simulink model "motorcontrol_codegen_19a"  (R2019a)
settings: Solver=FixedStepDiscrete  StartTime=0.0  StopTime=Inf  MaxStep=5e-5  RelTol=1e-3  EnableMultiTasking=on
values from neighbouring files (symbols this model uses):
  dataType = 'single'    [motorcontrol_codegen_params.m]
undefined symbols (not defined in the file or in its folder): ControlMode, ctrlParams, DiscIntNeverNeededParam, Down, GPTRIP1SEL, GPTRIP2SEL, inverter, mcb_isSimVar, NumBits1, NumBits2, PI_params, pmsm, Slope1, Slope2, Target, Ts, TZ1, TZ2, Up
libraries: simulink x14, c2802xlib x5, c2837xDlib x4, c280xlib x1, c2000lib x1
(part 1 of 3)
settings Model: SimulationMode=external  ExtModeTrigDuration=8  Creator=26046633  LastModifiedBy=26046633
settings SolverCC: ZeroCrossAlgorithm=Adaptive
settings OptimizationCC: DefaultUnderspecifiedDataType=single  StateBitsets=on  DataBitsets=on  NoFixptDivByZeroProtection=on  EfficientFloat2IntCast=on  LifeSpan=inf  MaxStackSize=1024  DifferentSizesBufferReuse=on  OptimizationPriority=RAM  DenormalBehavior=FlushToZero
settings DebuggingCC: IgnoredZcDiagnostic=none  MultiTaskDSMMsg=none  IntegerOverflowMsg=none  ParameterOverflowMsg=none  ParameterPrecisionLossMsg=none  ParameterTunabilityLossMsg=error
settings HardwareCC: ProdBitPerChar=16  ProdBitPerInt=16  ProdBitPerPointer=32  ProdBitPerSizeT=32  ProdBitPerPtrDiffT=32  ProdLargestAtomicInteger=Integer  ProdLargestAtomicFloat=None  ProdWordSize=16  ProdLongLongMode=on  ProdHWDeviceType=Texas Instruments->C2000
settings ModelReferenceCC: PropagateSignalLabelsOutOfModel=off
settings SFSimCC: MATLABDynamicMemAlloc=off
settings RTWCC: SystemTargetFile=ert.tlc  HardwareBoard=TI Delfino F2837xD  TLCOptions=-aInlineSetEventsForThisBaseRateFcn=TLC_FALSE -aSuppressMultiTaskScheduler=TLC_FALSE -aRateBasedStepFcn=1  GenCodeOnly=on  TemplateMakefile=ert_default_tmf  Toolchain=Texas Instruments Code Composer Studio (C2000)  PortableWordSizes=on  CreateSILPILBlock=SIL
settings CodeAppCC: ForceParamTrailComments=on  IgnoreCustomStorageClasses=off  OperatorAnnotations=on  SimulinkDataObjDesc=on  SFDataObjDesc=on  CustomSymbolStrGlobalVar=rt$N$M  CustomSymbolStrType=$N$M  CustomSymbolStrFcn=$N$M$F  CustomSymbolStrMacro=$N$M  InsertBlockDesc=on
settings ERTTargetCC: CodeReplacementLibrary=TI C28x  IncludeMdlTerminateFcn=off  CombineSignalStateStructs=on  SupportNonInlinedSFcns=on  ExtModeTransport=3  ExtModeStaticAllocSize=10000  ERTFilePackagingFormat=CompactWithDataFile

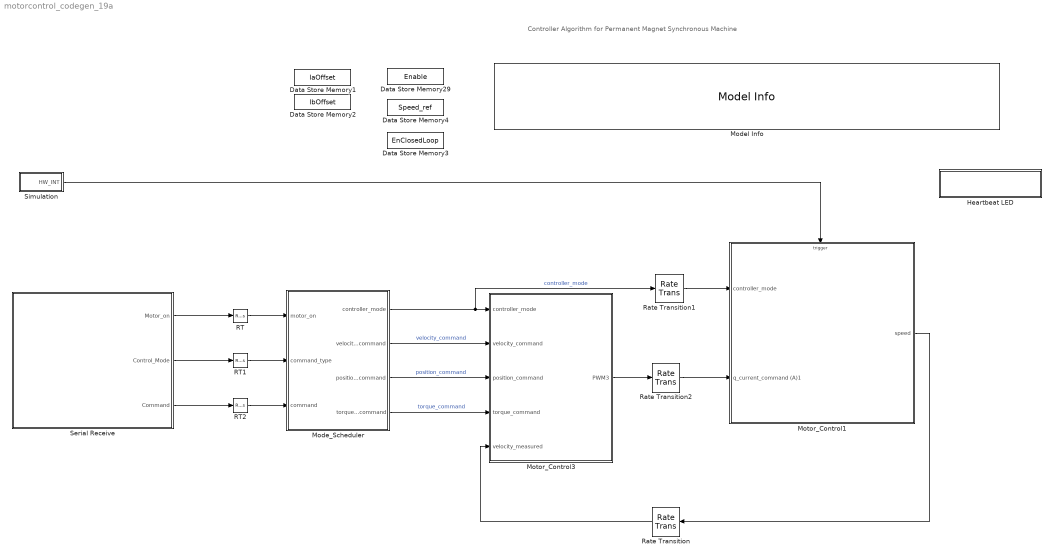
== system motorcontrol_codegen_19a ==
  note: Controller Algorithm for Permanent Magnet Synchronous Machine
  Data Store Memory1 : DataStoreMemory  DataStoreName=IaOffset  InitialValue=inverter.CtSensAOffset  ShowAdditionalParam=off
  Data Store Memory2 : DataStoreMemory  DataStoreName=IbOffset  InitialValue=inverter.CtSensBOffset  ShowAdditionalParam=off
  Data Store Memory29 : DataStoreMemory  DataStoreName=Enable  ShowAdditionalParam=off  OutDataTypeStr=boolean
  Data Store Memory3 : DataStoreMemory  DataStoreName=EnClosedLoop  ShowAdditionalParam=off  OutDataTypeStr=boolean
  Data Store Memory4 : DataStoreMemory  DataStoreName=Speed_ref  ShowAdditionalParam=off  OutDataTypeStr=dataType
  Heartbeat LED : Subsystem  TreatAsAtomicUnit=on
  Mode_Scheduler : Subsystem  TreatAsAtomicUnit=on  SystemSampleTime=Ts.speed
      mask Display: fprintf('Mode\nScheduler')
  Model Info : simulink/Model-Wide Utilities/Model Info  Frame=on  DisplayStringWithTags=|  HorizontalTextAlignment=Left  LeftAlignmentValue=0.02
      | %<Description>  Model Description: Controller Algorithm for Permanent Magnet Synchronous Motor
      | 
      | %<ModifiedComment> Specifies controller software for Permanent Magnet Synchronous Machine (PMSM) using Field-Oriented Control.
      | 
      | Created By: %<Created>  | Alper Senem [26046633]
      | Last Modification: %<LastModificationDate> | %<LastModifiedBy>
      | Version: %<ModelVersion>
  Motor_Control1 : Subsystem
      settings: RTWSystemCode=Nonreusable function
      mask Display: fprintf('Field Oriented\nControl')
  Motor_Control3 : Subsystem  TreatAsAtomicUnit=on  SystemSampleTime=Ts.speed
      settings: RTWSystemCode=Nonreusable function  RTWFcnNameOpts=Use subsystem name
      mask Display: fprintf('Motor\nControl')
  RT : RateTransition  Deterministic=off  OutPortSampleTime=Ts.speed
  RT1 : RateTransition  Integrity=off  Deterministic=off  OutPortSampleTime=Ts.speed
  RT2 : RateTransition  Deterministic=off  OutPortSampleTime=Ts.speed
  Rate Transition : RateTransition  Deterministic=off  OutPortSampleTime=Ts.speed
  Rate Transition1 : RateTransition  Integrity=off  Deterministic=off
  Rate Transition2 : RateTransition  Deterministic=off
  Serial Receive : Subsystem
  Simulation : Subsystem
  wires:
  RT1/1 -> Mode_Scheduler/2(command_type)
  RT2/1 -> Mode_Scheduler/3(command)
  Serial Receive/2(Control_Mode) -> RT1/1
  Rate Transition1/1 -> Motor_Control1/1(controller_mode)
  Motor_Control1/1(speed) -> Rate Transition/1
  Mode_Scheduler/2(velocity_command) -> Motor_Control3/2(velocity_command)  "velocity_command"
  Rate Transition2/1 -> Motor_Control1/2(q_current_command (A)1)
  Mode_Scheduler/3(position_command) -> Motor_Control3/3(position_command)  "position_command"
  Mode_Scheduler/4(torque_command) -> Motor_Control3/4(torque_command)  "torque_command"
  Mode_Scheduler/1(controller_mode) -> Motor_Control3/1(controller_mode), Rate Transition1/1  "controller_mode"
  Serial Receive/1(Motor_on) -> RT/1
  Simulation/1(HW_INT) -> Motor_Control1/Trigger
  Rate Transition/1 -> Motor_Control3/5(velocity_measured)
  RT/1 -> Mode_Scheduler/1(motor_on)
  Serial Receive/3(Command) -> RT2/1
  Motor_Control3/1(PWM3) -> Rate Transition2/1

== system motorcontrol_codegen_19a/Heartbeat LED ==
  note: Heartbeat LED 1HZ
  RED_LED : Constant  OutDataTypeStr=uint16  SampleTime=0.1
  Subsystem : Subsystem
  wires:
  RED_LED/1 -> Subsystem/1(In1)

== system motorcontrol_codegen_19a/Mode_Scheduler ==
  note: Mode Scheduler
  note: Configures controller mode and controller inputs based on user commands.
  motor_on : Inport
  command_type : Inport  Port=2
  command : Inport  Port=3
  Controller_Mode_Scheduler : Stateflow chart  SystemSampleTime=Ts
  Signal Conversion : SignalConversion  OverrideOpt=on
  Signal Conversion1 : SignalConversion  OverrideOpt=on
  Signal Conversion2 : SignalConversion  OverrideOpt=on
  controller_mode : Outport
  velocity_command : Outport  Port=2
  position_command : Outport  Port=3
  torque_command : Outport  Port=4
  wires:
  Signal Conversion2/1 -> Controller_Mode_Scheduler/3(command)
  Signal Conversion1/1 -> Controller_Mode_Scheduler/2(command_type)
  Signal Conversion/1 -> Controller_Mode_Scheduler/1(motor_on)
  command/1 -> Signal Conversion2/1
  Controller_Mode_Scheduler/4(torque_command) -> torque_command/1
  command_type/1 -> Signal Conversion1/1
  Controller_Mode_Scheduler/3(position_command) -> position_command/1
  motor_on/1 -> Signal Conversion/1
  Controller_Mode_Scheduler/2(velocity_command) -> velocity_command/1
  Controller_Mode_Scheduler/1(controller_mode) -> controller_mode/1

== system motorcontrol_codegen_19a/Motor_Control1 ==
  note: Field Oriented Controller
  note: This layer executes the control law, and calculates compare values used by the PWM driver.
      | The controller outputs compare values used by the Pulse Width Modulators (PWMs) to generate the phase voltages.
  controller_mode : Inport
  q_current_command (A)1 : Inport  Port=2
  Trigger : TriggerPort  TriggerType=function-call  VariantControl=Variant  SampleTime=-1  PortDimensions=1
  ControlSystem : Subsystem
  Demux1 : Demux
  Input Scaling : Subsystem
  "Inverter " : Subsystem
  Mux : Mux  Inputs=2
  Output Scaling : Subsystem
  Sensor Driver Blocks : Subsystem  VariantControl=mcb_isSimVar()
  speed : Outport
  wires:
  ControlSystem/1(Vabc) -> Output Scaling/1(Vabc_ref)
  Demux1/4 -> Input Scaling/4(QEP_Index_Latch)
  Output Scaling/2(PWM_Enable) -> Mux/2
  Input Scaling/3(EnClosedLoop) -> ControlSystem/5(EnClosedLoop)
  q_current_command (A)1/1 -> ControlSystem/2(q_current_command (A)1)
  Sensor Driver Blocks/1(Out) -> Demux1/1
  Input Scaling/2(Iab_meas) -> ControlSystem/4(Iab_fb)  "Iab_fb"
  Demux1/1 -> Input Scaling/1(Ia_ADC)
  Input Scaling/1(Pos) -> ControlSystem/3(Pos)  "Position"
  Input Scaling/4(speed) -> ControlSystem/6(speed), speed/1  "Speed"
  controller_mode/1 -> ControlSystem/1(controller_mode)
  Demux1/2 -> Input Scaling/2(Ib_ADC)
  Demux1/3 -> Input Scaling/3(QEP_Position_Count)
  Output Scaling/1(PWM_Duty_Cycles) -> Mux/1
  Mux/1 -> "Inverter "/1(Inverter Signals)

== system motorcontrol_codegen_19a/Motor_Control3 ==
  note: This layer executes the control law, and calculates compare values used by the PWM driver.
      | The controller outputs compare values used by the Pulse Width Modulators (PWMs) to generate the phase voltages.
  note: Motor Control
  controller_mode : Inport
  velocity_command : Inport  Port=2
  position_command : Inport  Port=3
  torque_command : Inport  Port=4
  velocity_measured : Inport  Port=5
  Control Modes : Subsystem
  Ground : Ground
  Rate Transition : RateTransition  Deterministic=off  OutPortSampleTime=Ts.speed
  Subsystem1 : Subsystem  mask{FilterConstant=0.01*(Ts.speed/Ts.pwm)}
      mask prompts: FilterConstant "Filter coefficient"
      mask help:
      | Implement an IIR Filter on target hardware by implementing the formula:
      |
      |  y_k = a.x_k + (1-a).y_(k-1)
      |
      | Where, a is the filter coefficient.
      | Lower filter coefficient gives better filtering, but increases the delay in response time.
      mask TypeOptions FilterConstant: Filter_Constant/Value
      mask DialogControl DescGroupVar Prompt: IIR Filter
      mask DialogControl DescTextVar Prompt: Implement an IIR Filter on target hardware by implementing the formula:   y_k = a.x_k + (1-a).y_(k-1)  Where, a is the filter coefficient. Lower filter coefficient gives better filtering, but increases the delay in response time.
      mask Display: fprintf('IIR\n Filter')
  Subsystem2 : Subsystem
  PWM3 : Outport
  wires:
  controller_mode/1 -> Control Modes/1(controller_mode)
  Control Modes/1(PWM3) -> PWM3/1
  Rate Transition/1 -> Control Modes/6(position_measured)
  position_command/1 -> Control Modes/5(position_command)
  torque_command/1 -> Control Modes/4(torque_command)
  Subsystem1/1(y) -> Control Modes/2(velocity_command)  "Speed_ref"
  velocity_command/1 -> Subsystem2/1(Speed_Ref_In)
  Subsystem2/1(Speed_Ref_PU) -> Subsystem1/1(x)  "Speed_Ref"
  velocity_measured/1 -> Subsystem2/2(Speed_Ref_Open), Control Modes/3(velocity_measured)  "Speed_fb"
  Ground/1 -> Rate Transition/1

== system motorcontrol_codegen_19a/Serial Receive ==
  Command_Type : simulink/Sources/Enumerated Constant  OutDataTypeStr=Enum: ControlMode  Value=ControlMode.Speed  SampleTime=-1
  Data Store Write : DataStoreWrite  DataStoreName=Enable
  Data Store Write1 : DataStoreWrite  DataStoreName=Speed_ref
  Data_Type_Float : Subsystem  VariantControl=isequal(dataType, 'single')
  Simulation : Subsystem
  unParse : Subsystem
  Motor_on : Outport
  Control_Mode : Outport  Port=2
  Command : Outport  Port=3
  wires:
  Data_Type_Float/1(Desired Speed) -> Data Store Write1/1, Command/1  "Command"
  Command_Type/1 -> Control_Mode/1  "Control_Mode"
  unParse/1(Enable_PWM) -> Motor_on/1, Data Store Write/1
  Data_Type_Float/2(Out2) -> unParse/1(Data)
  Simulation/1(Data) -> Data_Type_Float/1(Data)

== system motorcontrol_codegen_19a/Simulation ==
  C28x Hardware Interrupt : c2000lib/Scheduling/C28x Hardware Interrupt  irqnumbers=1  pienumbers=2  irqpriorities=30  irqpreempts=1  showinput=off  dspchiptype=C280X
      settings: SourceProductName=Embedded Coder Support Package for Texas Instruments C2000 Processors
  HW_INT : Outport
  wires:
  C28x Hardware Interrupt/1 -> HW_INT/1

== system motorcontrol_codegen_19a/Heartbeat LED/Subsystem ==
  In1 : Inport
  Digital Output : c2837xDlib/Digital Output  GPIO_Number=GPIO32~GPIO39  GPIO_Bit0=off  GPIO_BIT0_Toggle=on  GPIO_Bit1=off  GPIO_BIT1_Toggle=off  GPIO_Bit2=on  GPIO_BIT2_Toggle=on  GPIO_Bit3=off  GPIO_BIT3_Toggle=off  GPIO_Bit4=off  GPIO_BIT4_Toggle=off  GPIO_Bit5=off  GPIO_BIT5_Toggle=off  GPIO_Bit6=off  GPIO_BIT6_Toggle=off  GPIO_Bit7=off  GPIO_BIT7_Toggle=off
      settings: SourceProductName=Embedded Coder Support Package for Texas Instruments C2000 Processors
  wires:
  In1/1 -> Digital Output/1

== system motorcontrol_codegen_19a/Motor_Control1/ControlSystem ==
  controller_mode : Inport
  q_current_command (A)1 : Inport  Port=2
  Pos : Inport  Port=3
  Iab_fb : Inport  Port=4
  EnClosedLoop : Inport  Port=5
  speed : Inport  Port=6
  Closed_Loop : Subsystem
  NOT : Logic  Operator=NOT  IconShape=distinctive  AllPortsSameDT=off  OutDataTypeStr=boolean
  Open Loop Start-Up : Subsystem
  Switch4 : Switch  Threshold=0.5  OutDataTypeStr=Inherit: Inherit via back propagation  RndMeth=Simplest
  Vabc : Outport
  wires:
  Open Loop Start-Up/1(Vabc) -> Switch4/3
  EnClosedLoop/1 -> Closed_Loop/Enable, Switch4/2, NOT/1
  controller_mode/1 -> Closed_Loop/1(controller_mode)
  q_current_command (A)1/1 -> Closed_Loop/2(q_current_command (A)1)
  Closed_Loop/1(Vabc) -> Switch4/1
  NOT/1 -> Open Loop Start-Up/Enable
  Switch4/1 -> Vabc/1
  Pos/1 -> Closed_Loop/3(Feedback)
  Iab_fb/1 -> Closed_Loop/4(Iab_fb)
  speed/1 -> Closed_Loop/5(Speed)

== system motorcontrol_codegen_19a/Motor_Control1/Input Scaling ==
  note: QEP
  note: Position & Speed Measurements
  note: Current Measurements
  Ia_ADC : Inport
  Ib_ADC : Inport  Port=2
  QEP_Position_Count : Inport  Port=3
  QEP_Index_Latch : Inport  Port=4
  " Calculate Position and Speed" : Subsystem
  Calculate Phase Currents : Subsystem
  IndexOffset : Constant  Value=pmsm.PositionOffset * 2 * pi  OutDataTypeStr=dataType  SampleTime=-1
  Pos : Outport
  Iab_meas : Outport  Port=2
  EnClosedLoop : Outport  Port=3
  speed : Outport  Port=4
  wires:
  " Calculate Position and Speed"/3(IndexFound) -> EnClosedLoop/1
  IndexOffset/1 -> " Calculate Position and Speed"/3(Offset)
  QEP_Index_Latch/1 -> " Calculate Position and Speed"/2(QEP_Index_Latch)
  Ib_ADC/1 -> Calculate Phase Currents/2(Ib_ADC)
  Ia_ADC/1 -> Calculate Phase Currents/1(Ia_ADC)
  " Calculate Position and Speed"/1(Theta_e) -> Pos/1
  QEP_Position_Count/1 -> " Calculate Position and Speed"/1(QEP_Position_Count)
  Calculate Phase Currents/1(Iab_meas) -> Iab_meas/1  "Iab_fb"
  " Calculate Position and Speed"/2(speed) -> speed/1

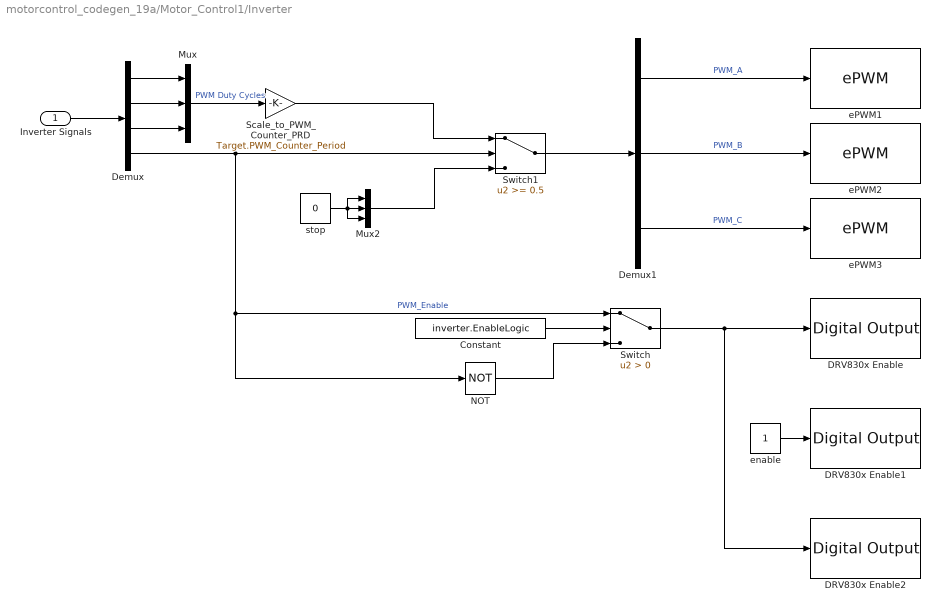
== system motorcontrol_codegen_19a/Motor_Control1/Inverter  ==
  Inverter Signals : Inport
  Constant : Constant  Value=inverter.EnableLogic  SampleTime=-1
  DRV830x Enable : c2837xDlib/Digital Output  GPIO_Number=GPIO40~GPIO47  GPIO_Bit0=on  GPIO_BIT0_Toggle=off  GPIO_Bit1=off  GPIO_BIT1_Toggle=off  GPIO_Bit2=off  GPIO_BIT2_Toggle=off  GPIO_Bit3=off  GPIO_BIT3_Toggle=off  GPIO_Bit4=off  GPIO_BIT4_Toggle=off  GPIO_Bit5=off  GPIO_BIT5_Toggle=off  GPIO_Bit6=off  GPIO_BIT6_Toggle=off  GPIO_Bit7=off  GPIO_BIT7_Toggle=off
      settings: SourceProductName=Embedded Coder Support Package for Texas Instruments C2000 Processors
  DRV830x Enable1 : c2837xDlib/Digital Output  GPIO_Number=GPIO40~GPIO47  GPIO_Bit0=off  GPIO_BIT0_Toggle=off  GPIO_Bit1=on  GPIO_BIT1_Toggle=off  GPIO_Bit2=off  GPIO_BIT2_Toggle=off  GPIO_Bit3=off  GPIO_BIT3_Toggle=off  GPIO_Bit4=off  GPIO_BIT4_Toggle=off  GPIO_Bit5=off  GPIO_BIT5_Toggle=off  GPIO_Bit6=off  GPIO_BIT6_Toggle=off  GPIO_Bit7=off  GPIO_BIT7_Toggle=off
      settings: SourceProductName=Embedded Coder Support Package for Texas Instruments C2000 Processors
  DRV830x Enable2 : c2837xDlib/Digital Output  GPIO_Number=GPIO56~GPIO63  GPIO_Bit0=off  GPIO_BIT0_Toggle=off  GPIO_Bit1=off  GPIO_BIT1_Toggle=off  GPIO_Bit2=on  GPIO_BIT2_Toggle=off  GPIO_Bit3=off  GPIO_BIT3_Toggle=off  GPIO_Bit4=off  GPIO_BIT4_Toggle=off  GPIO_Bit5=off  GPIO_BIT5_Toggle=off  GPIO_Bit6=off  GPIO_BIT6_Toggle=off  GPIO_Bit7=off  GPIO_BIT7_Toggle=off
      settings: SourceProductName=Embedded Coder Support Package for Texas Instruments C2000 Processors
  Demux : Demux
  Demux1 : Demux  Outputs=3
  Mux : Mux  Inputs=3
  Mux2 : Mux  Inputs=3
  NOT : Logic  Operator=NOT  IconShape=distinctive  AllPortsSameDT=off  OutDataTypeStr=boolean
  Scale_to_PWM_Counter_PRD : Gain  Gain=Target.PWM_Counter_Period  OutDataTypeStr=uint16  RndMeth=Simplest
  Switch : Switch  Criteria=u2 > Threshold  OutDataTypeStr=uint16
  Switch1 : Switch  Threshold=0.5
  ePWM1 : c2802xlib/ePWM  PwmType=C2000_Type4  useModule=ePWM1  ePWMxLINKTBPRD=Not Linked  periodUnits=Clock cycles  timerSource=Specify via dialog  timerPeriod_clk=Target.PWM_Counter_Period+1  timerPeriod_sec=0.0001  tbshadow=Immediate without using shadow  countingMode=Up-Down  phaseActiveEnable=Disable  phaseDirection=Count down after sync  phaseActive=0  synchronizationEnable=off  dcaevt1Sync=off  dcbevt1Sync=off  synchronizationOption=Counter equals to zero (CTR=Zero)  perSynchronizationOption=Counter equals to period (CTR=PRD)  clockPrescale=1  HSclockPrescale=1  enswap=off  ePWMxAStatus=on  ePWMxAactionLogic1=Do nothing  ePWMxAactionLogic2=Do nothing  ePWMxAactionLogic3=Clear  ePWMxAactionLogic4=Set  ePWMxAactionLogic5=Do nothing  ePWMxAactionLogic6=Do nothing  ePWMxACSFenable=off  ePWMxACSFvalue=Forcing disable  ePWMxASFreload=Zero  ePWMxBStatus=off  ePWMxBactionLogic1=Do nothing  ePWMxBactionLogic2=Do nothing  ePWMxBactionLogic3=Clear  ePWMxBactionLogic4=Set  ePWMxBactionLogic5=Do nothing  ePWMxBactionLogic6=Do nothing  ePWMxBCSFenable=off  ePWMxBCSFvalue=Forcing disable  ePWMxBSFreload=Zero  ePWNxBOutWay=off  ePWMxLINKCMPA=Not Linked  CMPAUnits=Clock cycles  CMPASource=Input port  CMPAValue_per=50  CMPAValue_clk=floor(Target.PWM_Counter_Period/2+1)  enCMPAshadow=Counter equals to zero (CTR=Zero)  ePWMxLINKCMPB=Not Linked  CMPBUnits=Clock cycles  CMPBSource=Specify via dialog  CMPBValue_per=50  CMPBValue_clk=floor(Target.PWM_Counter_Period/2+1)  enCMPBshadow=Counter equals to zero (CTR=Zero)  ePWMxLINKCMPC=Not Linked  CMPCUnits=Clock cycles  CMPCSource=Specify via dialog  CMPCValue_per=50  CMPCValue_clk=floor(Target.PWM_Counter_Period/2+1)  enCMPCshadow=Counter equals to zero (CTR=Zero)  ePWMxLINKCMPD=Not Linked  CMPDUnits=Clock cycles  CMPDSource=Specify via dialog  CMPDValue_per=50  CMPDValue_clk=floor(Target.PWM_Counter_Period/2+1)  enCMPDshadow=Counter equals to zero (CTR=Zero)  enableDBePWMxA=on  enableDBePWMxB=on  enhalfcycle=off  DBpolarity=Active high complementary (AHC)  DBedgeDelay=Positive  DBSource_ePWMxA=ePWMxA  DBSource_ePWMxB=ePWMxA  DBPeriodUnits=Clock cycles  DBperiodSource=Specify via dialog  REDperiod=200  FEDperiod=200  REDperiod_sec=0  FEDperiod_sec=0  LoadModeDBRED=Immediate without using shadow  LoadModeDBFED=Immediate without using shadow  adcstartModuleA=on  adcrequestEventA=First event  adcstartEventA=Digital Compare Module A Event 1 start of conversion (DCAEVT1.soc)  adcstartEventA_type2=Counter equals to period (CTR=PRD)  adcstartModuleB=off  adcrequestEventB=First event  adcstartEventB=Counter equals to zero (CTR=Zero)  adcstartEventB_type2=Counter equals to zero (CTR=Zero)  intEn=off  intPrd=First event  intSel=Counter equals to zero (CTR=Zero)  intSel_type2=Counter equals to zero (CTR=Zero)  hrpe=off  enHRPWM=off  HRPWM_LoadMode=Counter equals to period (CTR=PRD)  HRPWM_CTLMode=Duty or Period control mode  HRPWM_EDGMode=Both edge  hrpeb=off  enHRPWMB=off  HRPWM_LoadModeB=Counter equals to zero (CTR=ZERO)  HRPWM_CTLModeB=Duty or Period control mode  HRPWM_EDGModeB=Both edge  enHRDBRED=off  enHRDBFED=off  enSFO=on  enautoconv=on  chopperEnable=off  chopperFrequency=1  chopperFirstwidth=1  chopperDuty=12.5%  tripZonesource=Specify via dialog  tzselOSHT1=on  tzselOSHT2=off  tzselOSHT3=off  tzselOSHDCAEV1=on  tzselOSHDCBEV1=off  tzselCBC1=off  tzselCBC2=off  tzselCBC3=off  tzselCBCDCAEV2=off  tzselCBCDCBEV2=off  tzselOSHT4=off  tzselOSHT5=off  tzselOSHT6=off  tzselCBC4=off  tzselCBC5=off  tzselCBC6=off  enTzOstIntr=off  enTzCbcIntr=off  enTzDCAEVT1Intr=on  enTzDCAEVT2Intr=off  enTzDCBEVT1Intr=off  enTzDCBEVT2Intr=off  ePWMxAforced=Low  ePWMxBforced=Low  DCAEVT1forced=No action  DCBEVT1forced=No action  DCAEVT2forced=No action  DCBEVT2forced=No action  dcah=Trip Zone 1 input (TZ1)  dcal=Trip Zone 2 input (TZ2)  dcbh=Trip Zone 1 input (TZ1)  dcbl=Trip Zone 2 input (TZ2)  dcah_type2=GPTRIP4SEL  dcal_type2=GPTRIP4SEL  dcbh_type2=GPTRIP1SEL/(TZ1)  dcbl_type2=GPTRIP2SEL/(TZ2)  gendcaevt1=DCAH=high and DCAL=don't care  gendcaevt2=Event disabled  gendcbevt1=Event disabled  gendcbevt2=Event disabled  dcaevt1src=DCAEVT1 with async  dcaevt2src=DCAEVT2 with sync  dcbevt1src=DCBEVT1 with sync  dcbevt2src=DCBEVT2 with sync  pulsesel=Counter equals to zero (CTR=Zero)  blankinv=off  blankoffset=0  blankwidth=0  evsrcsel=Filtered version of DCAEVT1 (DCAEVT1FILT)  encape=off
      settings: SourceProductName=Embedded Coder Support Package for Texas Instruments C2000 Processors
  ePWM2 : c2802xlib/ePWM  PwmType=C2000_Type4  useModule=ePWM2  ePWMxLINKTBPRD=Not Linked  periodUnits=Clock cycles  timerSource=Specify via dialog  timerPeriod_clk=Target.PWM_Counter_Period+1  timerPeriod_sec=0.0001  tbshadow=Counter equals to zero  countingMode=Up-Down  phaseActiveEnable=Set counter to phase value specified via dialog  phaseDirection=Count up after sync  phaseActive=2  synchronizationEnable=off  dcaevt1Sync=off  dcbevt1Sync=off  synchronizationOption=Pass through (EPWMxSYNCI or SWFSYNC)  perSynchronizationOption=Counter equals to period (CTR=PRD)  clockPrescale=1  HSclockPrescale=1  enswap=off  ePWMxAStatus=on  ePWMxAactionLogic1=Do nothing  ePWMxAactionLogic2=Do nothing  ePWMxAactionLogic3=Clear  ePWMxAactionLogic4=Set  ePWMxAactionLogic5=Do nothing  ePWMxAactionLogic6=Do nothing  ePWMxACSFenable=off  ePWMxACSFvalue=Forcing disable  ePWMxASFreload=Zero  ePWMxBStatus=off  ePWMxBactionLogic1=Do nothing  ePWMxBactionLogic2=Do nothing  ePWMxBactionLogic3=Clear  ePWMxBactionLogic4=Set  ePWMxBactionLogic5=Do nothing  ePWMxBactionLogic6=Do nothing  ePWMxBCSFenable=off  ePWMxBCSFvalue=Forcing disable  ePWMxBSFreload=Zero  ePWNxBOutWay=off  ePWMxLINKCMPA=Not Linked  CMPAUnits=Clock cycles  CMPASource=Input port  CMPAValue_per=50  CMPAValue_clk=floor(Target.PWM_Counter_Period/2+1)  enCMPAshadow=Counter equals to zero (CTR=Zero)  ePWMxLINKCMPB=Not Linked  CMPBUnits=Clock cycles  CMPBSource=Specify via dialog  CMPBValue_per=50  CMPBValue_clk=floor(Target.PWM_Counter_Period/2+1)  enCMPBshadow=Counter equals to zero (CTR=Zero)  ePWMxLINKCMPC=Not Linked  CMPCUnits=Clock cycles  CMPCSource=Specify via dialog  CMPCValue_per=50  CMPCValue_clk=floor(Target.PWM_Counter_Period/2+1)  enCMPCshadow=Counter equals to zero (CTR=Zero)  ePWMxLINKCMPD=Not Linked  CMPDUnits=Clock cycles  CMPDSource=Specify via dialog  CMPDValue_per=50  CMPDValue_clk=floor(Target.PWM_Counter_Period/2+1)  enCMPDshadow=Counter equals to zero (CTR=Zero)  enableDBePWMxA=on  enableDBePWMxB=on  enhalfcycle=off  DBpolarity=Active high complementary (AHC)  DBedgeDelay=Positive  DBSource_ePWMxA=ePWMxA  DBSource_ePWMxB=ePWMxA  DBPeriodUnits=Clock cycles  DBperiodSource=Specify via dialog  REDperiod=200  FEDperiod=200  REDperiod_sec=0  FEDperiod_sec=0  LoadModeDBRED=Immediate without using shadow  LoadModeDBFED=Immediate without using shadow  adcstartModuleA=off  adcrequestEventA=First event  adcstartEventA=Digital Compare Module A Event 1 start of conversion (DCAEVT1.soc)  adcstartEventA_type2=Counter equals to period (CTR=PRD)  adcstartModuleB=off  adcrequestEventB=First event  adcstartEventB=Counter equals to zero (CTR=Zero)  adcstartEventB_type2=Counter equals to zero (CTR=Zero)  intEn=off  intPrd=First event  intSel=Counter equals to zero (CTR=Zero)  intSel_type2=Counter equals to zero (CTR=Zero)  hrpe=off  enHRPWM=off  HRPWM_LoadMode=Counter equals to period (CTR=PRD)  HRPWM_CTLMode=Duty or Period control mode  HRPWM_EDGMode=Both edge  hrpeb=off  enHRPWMB=off  HRPWM_LoadModeB=Counter equals to zero (CTR=ZERO)  HRPWM_CTLModeB=Duty or Period control mode  HRPWM_EDGModeB=Both edge  enHRDBRED=off  enHRDBFED=off  enSFO=on  enautoconv=on  chopperEnable=off  chopperFrequency=1  chopperFirstwidth=1  chopperDuty=12.5%  tripZonesource=Specify via dialog  tzselOSHT1=on  tzselOSHT2=off  tzselOSHT3=off  tzselOSHDCAEV1=on  tzselOSHDCBEV1=off  tzselCBC1=off  tzselCBC2=off  tzselCBC3=off  tzselCBCDCAEV2=off  tzselCBCDCBEV2=off  tzselOSHT4=off  tzselOSHT5=off  tzselOSHT6=off  tzselCBC4=off  tzselCBC5=off  tzselCBC6=off  enTzOstIntr=off  enTzCbcIntr=off  enTzDCAEVT1Intr=on  enTzDCAEVT2Intr=off  enTzDCBEVT1Intr=off  enTzDCBEVT2Intr=off  ePWMxAforced=Low  ePWMxBforced=Low  DCAEVT1forced=No action  DCBEVT1forced=No action  DCAEVT2forced=No action  DCBEVT2forced=No action  dcah=Trip Zone 1 input (TZ1)  dcal=Trip Zone 2 input (TZ2)  dcbh=Trip Zone 1 input (TZ1)  dcbl=Trip Zone 2 input (TZ2)  dcah_type2=GPTRIP4SEL  dcal_type2=GPTRIP4SEL  dcbh_type2=GPTRIP1SEL/(TZ1)  dcbl_type2=GPTRIP2SEL/(TZ2)  gendcaevt1=DCAH=high and DCAL=don't care  gendcaevt2=Event disabled  gendcbevt1=Event disabled  gendcbevt2=Event disabled  dcaevt1src=DCAEVT1 with async  dcaevt2src=DCAEVT2 with sync  dcbevt1src=DCBEVT1 with sync  dcbevt2src=DCBEVT2 with sync  pulsesel=Counter equals to zero (CTR=Zero)  blankinv=off  blankoffset=0  blankwidth=0  evsrcsel=Filtered version of DCAEVT1 (DCAEVT1FILT)  encape=off
      settings: SourceProductName=Embedded Coder Support Package for Texas Instruments C2000 Processors
  ePWM3 : c2802xlib/ePWM  PwmType=C2000_Type4  useModule=ePWM3  ePWMxLINKTBPRD=Not Linked  periodUnits=Clock cycles  timerSource=Specify via dialog  timerPeriod_clk=Target.PWM_Counter_Period+1  timerPeriod_sec=0.0001  tbshadow=Counter equals to zero or SYNC event  countingMode=Up-Down  phaseActiveEnable=Set counter to phase value specified via dialog  phaseDirection=Count up after sync  phaseActive=2  synchronizationEnable=off  dcaevt1Sync=off  dcbevt1Sync=off  synchronizationOption=Pass through (EPWMxSYNCI or SWFSYNC)  perSynchronizationOption=Counter equals to period (CTR=PRD)  clockPrescale=1  HSclockPrescale=1  enswap=off  ePWMxAStatus=on  ePWMxAactionLogic1=Do nothing  ePWMxAactionLogic2=Do nothing  ePWMxAactionLogic3=Clear  ePWMxAactionLogic4=Set  ePWMxAactionLogic5=Do nothing  ePWMxAactionLogic6=Do nothing  ePWMxACSFenable=off  ePWMxACSFvalue=Forcing disable  ePWMxASFreload=Zero  ePWMxBStatus=off  ePWMxBactionLogic1=Do nothing  ePWMxBactionLogic2=Do nothing  ePWMxBactionLogic3=Clear  ePWMxBactionLogic4=Set  ePWMxBactionLogic5=Do nothing  ePWMxBactionLogic6=Do nothing  ePWMxBCSFenable=off  ePWMxBCSFvalue=Forcing disable  ePWMxBSFreload=Zero  ePWNxBOutWay=off  ePWMxLINKCMPA=Not Linked  CMPAUnits=Clock cycles  CMPASource=Input port  CMPAValue_per=50  CMPAValue_clk=floor(Target.PWM_Counter_Period/2+1)  enCMPAshadow=Counter equals to zero (CTR=Zero)  ePWMxLINKCMPB=Not Linked  CMPBUnits=Clock cycles  CMPBSource=Specify via dialog  CMPBValue_per=50  CMPBValue_clk=floor(Target.PWM_Counter_Period/2+1)  enCMPBshadow=Counter equals to zero (CTR=Zero)  ePWMxLINKCMPC=Not Linked  CMPCUnits=Clock cycles  CMPCSource=Specify via dialog  CMPCValue_per=50  CMPCValue_clk=floor(Target.PWM_Counter_Period/2+1)  enCMPCshadow=Counter equals to zero (CTR=Zero)  ePWMxLINKCMPD=Not Linked  CMPDUnits=Clock cycles  CMPDSource=Specify via dialog  CMPDValue_per=50  CMPDValue_clk=floor(Target.PWM_Counter_Period/2+1)  enCMPDshadow=Counter equals to zero (CTR=Zero)  enableDBePWMxA=on  enableDBePWMxB=on  enhalfcycle=off  DBpolarity=Active high complementary (AHC)  DBedgeDelay=Positive  DBSource_ePWMxA=ePWMxA  DBSource_ePWMxB=ePWMxA  DBPeriodUnits=Clock cycles  DBperiodSource=Specify via dialog  REDperiod=200  FEDperiod=200  REDperiod_sec=0  FEDperiod_sec=0  LoadModeDBRED=Immediate without using shadow  LoadModeDBFED=Immediate without using shadow  adcstartModuleA=off  adcrequestEventA=First event  adcstartEventA=Digital Compare Module A Event 1 start of conversion (DCAEVT1.soc)  adcstartEventA_type2=Counter equals to period (CTR=PRD)  adcstartModuleB=off  adcrequestEventB=First event  adcstartEventB=Counter equals to zero (CTR=Zero)  adcstartEventB_type2=Counter equals to zero (CTR=Zero)  intEn=off  intPrd=First event  intSel=Counter equals to zero (CTR=Zero)  intSel_type2=Counter equals to zero (CTR=Zero)  hrpe=off  enHRPWM=off  HRPWM_LoadMode=Counter equals to period (CTR=PRD)  HRPWM_CTLMode=Duty or Period control mode  HRPWM_EDGMode=Both edge  hrpeb=off  enHRPWMB=off  HRPWM_LoadModeB=Counter equals to zero (CTR=ZERO)  HRPWM_CTLModeB=Duty or Period control mode  HRPWM_EDGModeB=Both edge  enHRDBRED=off  enHRDBFED=off  enSFO=on  enautoconv=on  chopperEnable=off  chopperFrequency=1  chopperFirstwidth=1  chopperDuty=12.5%  tripZonesource=Specify via dialog  tzselOSHT1=on  tzselOSHT2=off  tzselOSHT3=off  tzselOSHDCAEV1=on  tzselOSHDCBEV1=off  tzselCBC1=off  tzselCBC2=off  tzselCBC3=off  tzselCBCDCAEV2=off  tzselCBCDCBEV2=off  tzselOSHT4=off  tzselOSHT5=off  tzselOSHT6=off  tzselCBC4=off  tzselCBC5=off  tzselCBC6=off  enTzOstIntr=off  enTzCbcIntr=off  enTzDCAEVT1Intr=on  enTzDCAEVT2Intr=off  enTzDCBEVT1Intr=off  enTzDCBEVT2Intr=off  ePWMxAforced=Low  ePWMxBforced=Low  DCAEVT1forced=No action  DCBEVT1forced=No action  DCAEVT2forced=No action  DCBEVT2forced=No action  dcah=Trip Zone 1 input (TZ1)  dcal=Trip Zone 2 input (TZ2)  dcbh=Trip Zone 1 input (TZ1)  dcbl=Trip Zone 2 input (TZ2)  dcah_type2=GPTRIP4SEL  dcal_type2=GPTRIP4SEL  dcbh_type2=GPTRIP1SEL/(TZ1)  dcbl_type2=GPTRIP2SEL/(TZ2)  gendcaevt1=DCAH=high and DCAL=don't care  gendcaevt2=Event disabled  gendcbevt1=Event disabled  gendcbevt2=Event disabled  dcaevt1src=DCAEVT1 with async  dcaevt2src=DCAEVT2 with sync  dcbevt1src=DCBEVT1 with sync  dcbevt2src=DCBEVT2 with sync  pulsesel=Counter equals to zero (CTR=Zero)  blankinv=off  blankoffset=0  blankwidth=0  evsrcsel=Filtered version of DCAEVT1 (DCAEVT1FILT)  encape=off
      settings: SourceProductName=Embedded Coder Support Package for Texas Instruments C2000 Processors
  enable : Constant  OutDataTypeStr=uint16  SampleTime=-1
  stop : Constant  Value=0  OutDataTypeStr=uint16  SampleTime=-1
  wires:
  stop/1 -> Mux2/3, Mux2/2, Mux2/1
  Inverter Signals/1 -> Demux/1
  Demux1/3 -> ePWM3/1  "PWM_C"
  Switch1/1 -> Demux1/1
  Scale_to_PWM_Counter_PRD/1 -> Switch1/1
  Mux/1 -> Scale_to_PWM_Counter_PRD/1  "PWM Duty Cycles"
  Demux1/2 -> ePWM2/1  "PWM_B"
  Demux/1 -> Mux/1
  Demux/2 -> Mux/2
  Demux/3 -> Mux/3
  Demux1/1 -> ePWM1/1  "PWM_A"
  Mux2/1 -> Switch1/3
  Constant/1 -> Switch/2
  Demux/4 -> Switch1/2, Switch/1, NOT/1  "PWM_Enable"
  NOT/1 -> Switch/3
  enable/1 -> DRV830x Enable1/1
  Switch/1 -> DRV830x Enable2/1, DRV830x Enable/1

== system motorcontrol_codegen_19a/Motor_Control1/Output Scaling ==
  Vabc_ref : Inport  OutDataTypeStr=dataType
  Constant : Constant  Value=0.5  OutDataTypeStr=dataType  SampleTime=-1
  Data Type Conversion : DataTypeConversion  OutDataTypeStr=dataType
  Enable : DataStoreRead  DataStoreName=Enable
  One_by_Two : Gain  Gain=1/ (2 * inverter.V_dc)  OutDataTypeStr=dataType  RndMeth=Simplest
  Sum : Sum  Inputs=|++  OutDataTypeStr=dataType
  PWM_Duty_Cycles : Outport  OutDataTypeStr=dataType
  PWM_Enable : Outport  Port=2
  wires:
  One_by_Two/1 -> Sum/1
  Sum/1 -> PWM_Duty_Cycles/1  "PWM_Duty_Cycles"
  Vabc_ref/1 -> One_by_Two/1
  Constant/1 -> Sum/2
  Enable/1 -> Data Type Conversion/1  "PWM_En"
  Data Type Conversion/1 -> PWM_Enable/1

== system motorcontrol_codegen_19a/Motor_Control1/Sensor Driver Blocks ==
  ADC_A_IN2 : c2802xlib/ADC  blkParamProc=C2000_Type4  ADCModule=A  samplingMode=Single sample mode  ADCResolution=12-bit (Single-ended input)  useSOC1=SOC1  useSOC2=SOC0_SOC1  SOCAcquisitionWindow=31  SOCTriggerSource=ePWM1_ADCSOCA  SOCInterruptTrigger=No ADCINT  Ts=-1  dType=uint16  postInterrupt=off  interruptSel=ADCINT1  ADCINTContinuous=on  endma=off  chdma=1  conv1=ADCINA0  conv2=ADCINA0 and ADCINB0  conv1_Type4=ADCIN2  conv2_Type4=ADCIN0 and ADCIN1
      settings: SourceProductName=Embedded Coder Support Package for Texas Instruments C2000 Processors
  ADC_B_IN2 : c2802xlib/ADC  blkParamProc=C2000_Type4  ADCModule=B  samplingMode=Single sample mode  ADCResolution=12-bit (Single-ended input)  useSOC1=SOC1  useSOC2=SOC0_SOC1  SOCAcquisitionWindow=31  SOCTriggerSource=ePWM1_ADCSOCA  SOCInterruptTrigger=No ADCINT  Ts=-1  dType=uint16  postInterrupt=on  interruptSel=ADCINT1  ADCINTContinuous=on  endma=off  chdma=1  conv1=ADCINA0  conv2=ADCINA0 and ADCINB0  conv1_Type4=ADCIN2  conv2_Type4=ADCIN0 and ADCIN1
      settings: SourceProductName=Embedded Coder Support Package for Texas Instruments C2000 Processors
  Mux1 : Mux
  eQEP : c280xlib/eQEP  useModule=eQEP1  pcInputmode=Quadrature-count  externalClockrate=2x resolution: Count the rising/falling edge  swapPolarityselection=Clockwise  qdfOutputport=off  qapPolarityselection=on  qbpPolarityselection=on  qipPolarityselection=on  qspPolarityselection=off  igatePolarityselection=off  sampleTime=-1  pcOutputport=on  pcMaximumvalue=2^16-1  indexInitializationcheck=off  indexInitializationevent=Rising edge  strobeInitializationcheck=off  strobeInitializationevent=Rising edge  softwareInitializationcheck=off  softwareInitializationsource=Set to init value at start up  softwareInitializationmode=on  pcInitialvalue=2147483648  pcResetmode=Reset on the first index event  ieloutputport=on  indexEventlatch=Falling edge  seloutputport=off  strobeEventlatch=Rising edge  pcefOutputport=off  enableEqepcapture=off  qctmrOutputport=off  qcprdOutputport=off  captureTimerprescaler=128  upEventprescaler=128  overflowErrorflag=off  directionErrorflag=off  captureTimerposition=On position counter read  unitTimerperiod=100000000  captureTimerlatch=off  capturePeriodlatch=off  positionCounterlatch=off  soenPolarityselection=off  spselPolarityselection=Index pin is used for sync output  compareValuesource=Specify via dialog  shadowMode=Load on QPOSCNT=0  compareValue=4294967295  syncOutputwidth=1  polaritySyncoutput=Active high  watchdogEnable=off  watchdogTimer=65535  outport1Datatype=auto  outport2Datatype=auto  outport3Datatype=auto  outport4Datatype=auto  outport5Datatype=auto  outport6Datatype=auto  outport7Datatype=auto  outport8Datatype=auto  outport9Datatype=auto  outport10Datatype=auto  outport11Datatype=auto  outport12Datatype=auto  eqepinterrupt_pce=off  eqepinterrupt_qpe=off  eqepinterrupt_qdc=off  eqepinterrupt_wto=off  eqepinterrupt_pcu=off  eqepinterrupt_pco=off  eqepinterrupt_pcr=off  eqepinterrupt_pcm=off  eqepinterrupt_sel=off  eqepinterrupt_iel=off  eqepinterrupt_uto=off  pheOutputport=off  watchdogOutputport=off  outport13Datatype=auto  outport14Datatype=auto
      settings: SourceProductName=Embedded Coder Support Package for Texas Instruments C2000 Processors
  Out : Outport
  wires:
  ADC_B_IN2/1 -> Mux1/2
  Mux1/1 -> Out/1
  eQEP/2 -> Mux1/4
  eQEP/1 -> Mux1/3
  ADC_A_IN2/1 -> Mux1/1

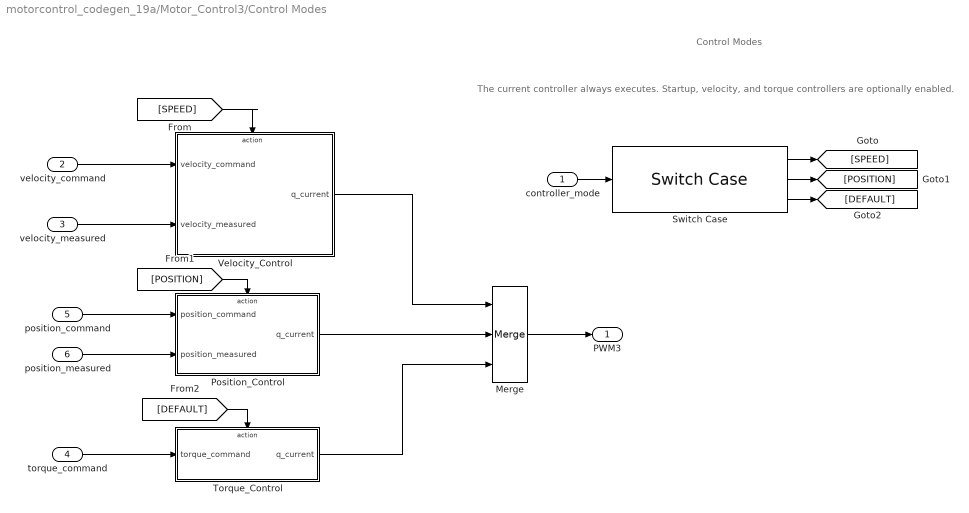
== system motorcontrol_codegen_19a/Motor_Control3/Control Modes ==
  note: The current controller always executes. Startup, velocity, and torque controllers are optionally enabled.
  note: Control Modes
  controller_mode : Inport
  velocity_command : Inport  Port=2
  velocity_measured : Inport  Port=3
  torque_command : Inport  Port=4
  position_command : Inport  Port=5
  position_measured : Inport  Port=6
  Merge : Merge  Inputs=3
  Position_Control : Subsystem  TreatAsAtomicUnit=on
  Switch Case : SwitchCase  CaseConditions={ControllerMode.SpeedControl,ControllerMode.PositionControl}
  Torque_Control : Subsystem  TreatAsAtomicUnit=on
  Velocity_Control : Subsystem
  PWM3 : Outport
  wires:
  velocity_measured/1 -> Velocity_Control/2(velocity_measured)
  Position_Control/1(q_current) -> Merge/2
  Velocity_Control/1(q_current) -> Merge/1
  Torque_Control/1(q_current) -> Merge/3
  torque_command/1 -> Torque_Control/1(torque_command)
  position_command/1 -> Position_Control/1(position_command)
  Switch Case/1 -> [SPEED]
  Switch Case/2 -> [POSITION]
  Switch Case/3 -> [DEFAULT]
  [SPEED] -> Velocity_Control/Action
  [POSITION] -> Position_Control/Action
  [DEFAULT] -> Torque_Control/Action
  position_measured/1 -> Position_Control/2(position_measured)
  velocity_command/1 -> Velocity_Control/1(velocity_command)
  controller_mode/1 -> Switch Case/1
  Merge/1 -> PWM3/1

== system motorcontrol_codegen_19a/Motor_Control3/Subsystem1 ==
  x : Inport
  Add : Sum
  Add1 : Sum  Inputs=-+
  Constant : Constant  OutDataTypeStr=dataType  SampleTime=-1
  Data Type Duplicate : DataTypeDuplicate  NumInputPorts=3
  Filter_Constant : Constant  Value=FilterConstant  OutDataTypeStr=dataType  SampleTime=-1
  Product : Product
  Product1 : Product
  Unit Delay : UnitDelay  SampleTime=-1  HasFrameUpgradeWarning=on
  y : Outport
  wires:
  x/1 -> Product/1, Data Type Duplicate/1
  Filter_Constant/1 -> Product/2, Add1/1, Data Type Duplicate/2
  Product/1 -> Add/1
  Add/1 -> y/1, Unit Delay/1
  Product1/1 -> Add/2
  Unit Delay/1 -> Product1/2
  Add1/1 -> Product1/1
  Constant/1 -> Data Type Duplicate/3, Add1/2

== system motorcontrol_codegen_19a/Motor_Control3/Subsystem2 ==
  Speed_Ref_In : Inport
  Speed_Ref_Open : Inport  Port=2
  AND : Logic  IconShape=distinctive  AllPortsSameDT=off  OutDataTypeStr=boolean
  Data Store Read : DataStoreRead  DataStoreName=EnClosedLoop
  Data Store Read1 : DataStoreRead  DataStoreName=Enable
  RPM to rad/s : Gain  Gain=2 * pi / 60  RndMeth=Simplest  OutDataTypeStr=Inherit: Same as input
  Switch : Switch  Criteria=u2 > Threshold  Threshold=0.5  OutDataTypeStr=single
  Speed_Ref_PU : Outport
  wires:
  RPM to rad/s/1 -> Switch/1
  Data Store Read1/1 -> AND/2
  Switch/1 -> Speed_Ref_PU/1
  Speed_Ref_Open/1 -> Switch/3
  Speed_Ref_In/1 -> RPM to rad/s/1
  Data Store Read/1 -> AND/1
  AND/1 -> Switch/2

== system motorcontrol_codegen_19a/Serial Receive/Data_Type_Float ==
  Data : Inport
  Data Type Conversion2 : DataTypeConversion  OutDataTypeStr=uint16  RndMeth=Simplest
  Demux : Demux  Outputs=2
  Desired Speed : Outport
  Out2 : Outport  Port=2
  wires:
  Demux/2 -> Data Type Conversion2/1
  Data Type Conversion2/1 -> Out2/1
  Demux/1 -> Desired Speed/1
  Data/1 -> Demux/1

== system motorcontrol_codegen_19a/Serial Receive/Simulation ==
  Data Type Conversion2 : DataTypeConversion  OutDataTypeStr=dataType  RndMeth=Simplest
  Data_Type_Float : Subsystem  VariantControl=isequal(dataType, 'single')
  Enable : Constant  OutDataTypeStr=uint16  SampleTime=-1
  Parse : Subsystem
  Speed_Ref_Final (rpm) : Constant  Value=100  OutDataTypeStr=dataType  SampleTime=-1
  Data : Outport
  wires:
  Data Type Conversion2/1 -> Data_Type_Float/1(In1)
  Speed_Ref_Final (rpm)/1 -> Data Type Conversion2/1
  Parse/1(Data) -> Data_Type_Float/2(In2)
  Enable/1 -> Parse/1(Enable_PWM)
  Data_Type_Float/1(Data) -> Data/1

== system motorcontrol_codegen_19a/Serial Receive/unParse ==
  Data : Inport
  Bitwise Operator : simulink/Logic and Bit Operations/Bitwise Operator  logicop=AND  UseBitMask=on  BitMask=hex2dec('0001')  BitMaskRealWorld=Stored Integer
  Data Type Conversion3 : DataTypeConversion  OutDataTypeStr=boolean  RndMeth=Simplest
  Enable_PWM : Outport
  wires:
  Data Type Conversion3/1 -> Enable_PWM/1
  Bitwise Operator/1 -> Data Type Conversion3/1
  Data/1 -> Bitwise Operator/1

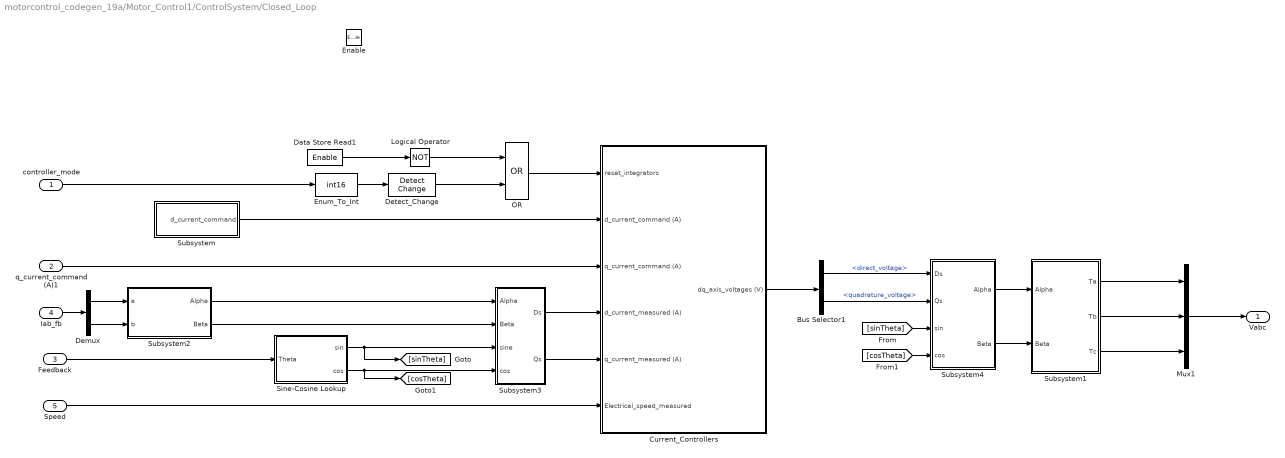
== system motorcontrol_codegen_19a/Motor_Control1/ControlSystem/Closed_Loop ==
  controller_mode : Inport
  q_current_command (A)1 : Inport  Port=2
  Feedback : Inport  Port=3
  Iab_fb : Inport  Port=4
  Speed : Inport  Port=5
  Enable : EnablePort  StatesWhenEnabling=reset
  Bus Selector1 : BusSelector  OutputSignals=direct_voltage,quadrature_voltage
  Current_Controllers : Subsystem  Description=|
      | Linear Current Controllers
      | 
      | PID Blocks used for Control Design of Current Loop controllers.
  Data Store Read1 : DataStoreRead  DataStoreName=Enable
  Demux : Demux  Outputs=2
  Detect_Change : simulink/Logic and Bit Operations/Detect Change  vinit=0  OutDataTypeStr=uint8
  Enum_To_Int : DataTypeConversion  OutDataTypeStr=int16
  Logical Operator : Logic  Operator=NOT  IconShape=distinctive  AllPortsSameDT=off  OutDataTypeStr=boolean
  Mux1 : Mux  Inputs=3
  OR : Logic  Operator=OR  AllPortsSameDT=off  OutDataTypeStr=boolean
  Sine-Cosine Lookup : Subsystem  mask{N_points=1024}
      mask prompts: N_points "Number of data points for lookup table:"
      mask init:
      | this = get_param(gcbh,'Object');
      | 
      | points = eval(this.N_points);
      | 
      | dlgSett.points = 125*floor(points/125);
      | 
      | dlgSett.Offset = uint16(dlgSett.points/5);
      | 
      | dlgSett.N_points = 4*dlgSett.Offset;
      | N_points = dlgSett.N_points;
      | 
      | theta = linspace(0,2*pi,N_points+1);
      | dlgSett.size = 5*dlgSett.Offset+2;
      | dlgSett.sin_table = zeros(1,dlgSett.size);
      | dlgSett.sin_table(1:N_points+1) = sin(theta);
      | dlgSett.sin_table(N_points+2:dlgSett.size) = dlgSett.sin_table(2:0.25*N_points+2);
      | 
      | dlgSett.N_points = double(dlgSett.N_points);
      | dlgSett.index_gain = dlgSett.N_points;
      | dlgSett.UpperSatLimit = 1;
      | dlgSett.UpperSatLimit = 2*pi;
      mask DialogControl DescGroupVar Prompt: Sine-Cosine Lookup
      mask DialogControl DescTextVar Prompt: Implement sine and cosine functions using a lookup table approach for optimized performance on target hardware.
      mask Display: fprintf('Sin-Cos\n LUT');
  Subsystem : Subsystem
  Subsystem1 : Subsystem  mask(Space Vector Generator){}
      mask help:
      | <p>Generate space vector modulation signals from stator reference voltages described by  &alpha;-&beta; components.
      | <br><br>
      | The block accepts V<sub>&alpha;</sub> and V<sub>&beta;</sub> voltages and outputs corresponding space vector modulation voltages.</p>
      mask Display: fprintf('Space\n Vector\n Generation');
  Subsystem2 : Subsystem  mask(Clarke Transform){}
      mask help:
      | <p>Compute Clarke transformation on balanced 3-phase inputs into balanced 2-phase orthogonal outputs.
      | <br>
      | <br>
      | The block accepts two signals out of three phases, and outputs corresponding &alpha;-&beta; axis components, where phase-a axis is aligned with alpha axis.</p>
      mask Display: fprintf('Clarke\nTransform');
  Subsystem3 : Subsystem  mask(Park Transform){AxisAlignment=D-axis}
      mask prompts: AxisAlignment "Alpha (phase-a) axis alignment:"
      mask help:
      | <p>Compute Park transformation on stationary reference frame inputs into rotating reference frame outputs.
      | <br><br>
      | The block accepts the following:
      | <ul>
      |   <li>&alpha;-&beta; axis components in stationary reference frame</li>
      |   <li>Sine and cosine values of corresponding angle of transformation</li>
      | </ul>
      | The block outputs direct and quadrature axis components in rotating reference frame.
      | <br><br>
      | D-axis alignment with alpha (phase-a) is popular in motor control theory while Q-axis alignment with alpha (phase-a) is more suitable for power conversion applications.</p>
      mask init:
      | dlgSett.Offset = 0;
      | 
      | switch AxisAlignment
      |     case 'Q-axis'
      |         dlgSett.Offset = 90;
      |     case 'D-axis'
      |         dlgSett.Offset = 0;
      |     otherwise
      | end
      mask TypeOptions AxisAlignment: D-axis | Q-axis
      mask Display: fprintf('Park\nTransform');
  Subsystem4 : Subsystem  mask(Inverse Park Transform){AxisAlignment=D-axis}
      mask prompts: AxisAlignment "Alpha (phase-a ) axis alignment:"
      mask help:
      | <p>Compute Inverse Park transformation on rotating reference frame inputs into stationary reference frame outputs.
      | <br><br>
      | The block accepts the following:
      | <ul>
      | <li>d-q axis components in rotating reference frame</li>
      | <li>Sine and cosine values of corresponding angle of transformation</li>
      | </ul>
      | The block outputs &alpha;-&beta; axis components in stationary reference frame.
      | <br><br>
      | D-axis alignment with alpha (phase-a) is popular in motor control theory while Q-axis alignment with alpha (phase-a) is more suitable for power conversion applications.</p>
      mask init:
      | dlgSett.Offset = 0;
      | 
      | switch AxisAlignment
      |     case 'Q-axis'
      |         dlgSett.Offset = 90;
      |     case 'D-axis'
      |         dlgSett.Offset = 0;
      |     otherwise
      | end
      mask TypeOptions AxisAlignment: D-axis | Q-axis
      mask Display: fprintf('Inverse Park\n Transform');
  Vabc : Outport
  wires:
  Subsystem3/2(Qs) -> Current_Controllers/5(q_current_measured (A))
  Sine-Cosine Lookup/1(sin) -> [sinTheta], Subsystem3/3(sine)
  Subsystem1/2(Tb) -> Mux1/2
  Demux/2 -> Subsystem2/2(b)
  Subsystem4/2(Beta) -> Subsystem1/2(Beta)
  [cosTheta] -> Subsystem4/4(cos)
  Subsystem/1(d_current_command) -> Current_Controllers/2(d_current_command (A))
  Sine-Cosine Lookup/2(cos) -> [cosTheta], Subsystem3/4(cos)
  Bus Selector1/2 -> Subsystem4/2(Qs)  "<quadrature_voltage>"
  Enum_To_Int/1 -> Detect_Change/1
  Subsystem4/1(Alpha) -> Subsystem1/1(Alpha)
  controller_mode/1 -> Enum_To_Int/1
  q_current_command (A)1/1 -> Current_Controllers/3(q_current_command (A))
  Iab_fb/1 -> Demux/1
  Data Store Read1/1 -> Logical Operator/1
  Mux1/1 -> Vabc/1
  Current_Controllers/1(dq_axis_voltages (V)) -> Bus Selector1/1
  Speed/1 -> Current_Controllers/6(Electrical_speed_measured)
  Subsystem3/1(Ds) -> Current_Controllers/4(d_current_measured (A))
  Subsystem1/1(Ta) -> Mux1/1
  Detect_Change/1 -> OR/2
  Bus Selector1/1 -> Subsystem4/1(Ds)  "<direct_voltage>"
  Logical Operator/1 -> OR/1
  Subsystem1/3(Tc) -> Mux1/3
  OR/1 -> Current_Controllers/1(reset_integrators)
  [sinTheta] -> Subsystem4/3(sin)
  Demux/1 -> Subsystem2/1(a)
  Subsystem2/2(Beta) -> Subsystem3/2(Beta)
  Subsystem2/1(Alpha) -> Subsystem3/1(Alpha)
  Feedback/1 -> Sine-Cosine Lookup/1(Theta)

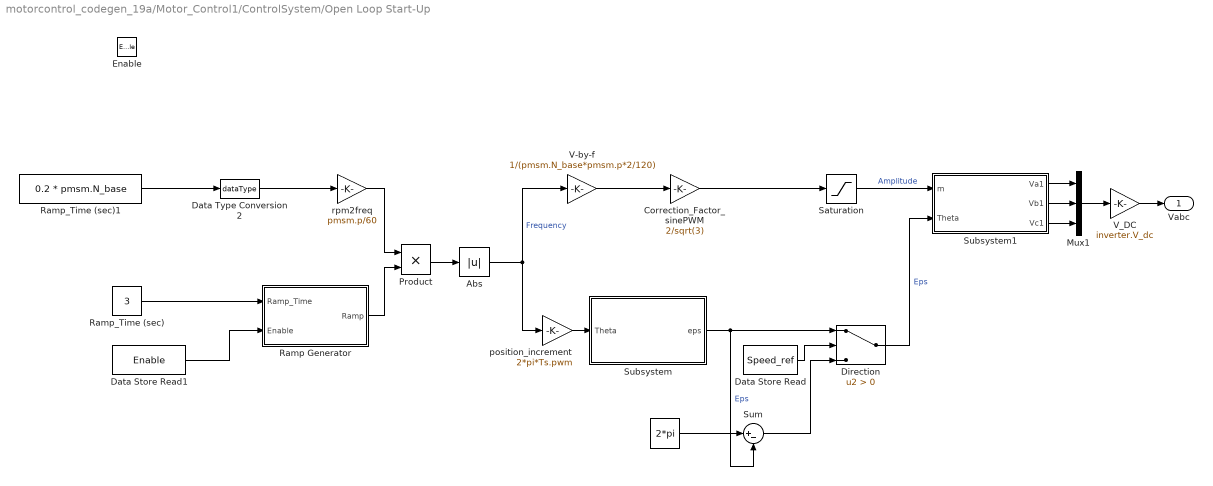
== system motorcontrol_codegen_19a/Motor_Control1/ControlSystem/Open Loop Start-Up ==
  Enable : EnablePort  StatesWhenEnabling=reset
  " " : Constant  Value=2*pi  OutDataTypeStr=dataType  SampleTime=-1
  Abs : Abs
  Correction_Factor_sinePWM : Gain  Gain=2/sqrt(3)  RndMeth=Simplest  OutDataTypeStr=Inherit: Same as input
  Data Store Read : DataStoreRead  DataStoreName=Speed_ref
  Data Store Read1 : DataStoreRead  DataStoreName=Enable
  Data Type Conversion2 : DataTypeConversion  OutDataTypeStr=dataType  RndMeth=Simplest
  Direction : Switch  Criteria=u2 > Threshold  OutDataTypeStr=dataType  RndMeth=Simplest
  Mux1 : Mux  Inputs=3
  Product : Product  RndMeth=Simplest  OutDataTypeStr=Inherit: Same as first input
  Ramp Generator : Subsystem
  Ramp_Time (sec) : Constant  Value=3  OutDataTypeStr=dataType  SampleTime=-1
  Ramp_Time (sec)1 : Constant  Value=0.2 * pmsm.N_base  OutDataTypeStr=dataType  SampleTime=-1
  Saturation : Saturate  UpperLimit=0.95  LowerLimit=0.15  RndMeth=Simplest
  Subsystem : Subsystem  mask(Position Generator){Offset=0, InitialCondition=0}
      mask prompts: Offset "Initial Theta output:"; InitialCondition "Initial condition"
      mask help:
      | <p>Generate position ramp of required frequency.
      | <br><br>
      | The block accepts position increment and outputs position ramp.
      | <br>
      | The position increment for required frequency (Hz) can be computed by following:
      | <br><br>
      | &Delta;&theta; (per-unit) = Frequency&#8231;Sample Time
      | <br>
      | &Delta;&theta; (radians)&nbsp; = 2&#8231;&pi;&#8231;Frequency&#8231;Sample Time
      | <br>
      | &Delta;&theta; (degrees) = 360&#8231;Frequency&#8231;Sample Time <br>
      mask Display: fprintf('Position\n Generator');
  Subsystem1 : Subsystem  mask(3-Phase Sine Voltage Generator){}
      mask help:
      | Generate balanced 3-phase sinusoidal signals described by magnitude and position inputs.
      |
      | The block accepts voltage reference by magnitude and position inputs, and outputs balanced three phase sinusoidal voltages of frequency corresponding to position input.
      |
      | Enter position input units and number of data points for sine-cosine look-up table.
      mask Display: fprintf('3-Phase Sine\n  Voltage Generator');
  Sum : Sum  Inputs=|+-  RndMeth=Simplest  OutDataTypeStr=Inherit: Same as first input
  V-by-f : Gain  Gain=1/(pmsm.N_base*pmsm.p*2/120)  RndMeth=Simplest  OutDataTypeStr=Inherit: Same as input
  V_DC : Gain  Gain=inverter.V_dc
  position_increment : Gain  Gain=2*pi*Ts.pwm  RndMeth=Simplest  OutDataTypeStr=Inherit: Same as input
  rpm2freq : Gain  Gain=pmsm.p/60  RndMeth=Simplest  OutDataTypeStr=Inherit: Same as input
  Vabc : Outport  VectorParamsAs1DForOutWhenUnconnected=off
  wires:
  V_DC/1 -> Vabc/1
  Data Store Read/1 -> Direction/2
  Ramp_Time (sec)1/1 -> Data Type Conversion2/1
  Data Type Conversion2/1 -> rpm2freq/1
  Correction_Factor_sinePWM/1 -> Saturation/1
  Data Store Read1/1 -> Ramp Generator/2(Enable)
  rpm2freq/1 -> Product/1
  Product/1 -> Abs/1
  V-by-f/1 -> Correction_Factor_sinePWM/1
  position_increment/1 -> Subsystem/1(Theta)
  Abs/1 -> V-by-f/1, position_increment/1  "Frequency"
  Sum/1 -> Direction/3
  " "/1 -> Sum/1
  Subsystem/1(eps) -> Direction/1, Sum/2  "Eps"
  Ramp_Time (sec)/1 -> Ramp Generator/1(Ramp_Time)
  Ramp Generator/1(Ramp) -> Product/2
  Mux1/1 -> V_DC/1
  Saturation/1 -> Subsystem1/1(m)  "Amplitude"
  Direction/1 -> Subsystem1/2(Theta)  "Eps"
  Subsystem1/2(Vb1) -> Mux1/2
  Subsystem1/1(Va1) -> Mux1/1
  Subsystem1/3(Vc1) -> Mux1/3
